simulink model "simulation"  (R2018a)
settings: Solver=VariableStepAuto  StartTime=0.0  StopTime=10.0  RelTol=1e-3
undefined symbols (not defined in the file or in its folder): booleanControl
settings Model: Creator=daniel  LastModifiedBy=daniel

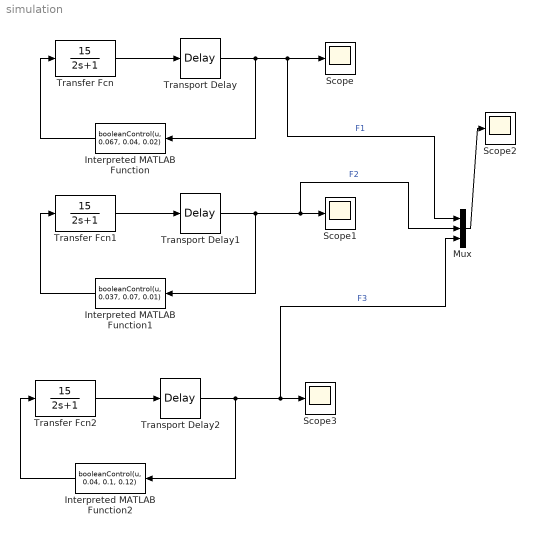
== system simulation ==
  Interpreted MATLAB Function : MATLABFcn  MATLABFcn=booleanControl(u, 0.067, 0.04, 0.02)
  Interpreted MATLAB Function1 : MATLABFcn  MATLABFcn=booleanControl(u, 0.037, 0.07, 0.01)
  Interpreted MATLAB Function2 : MATLABFcn  MATLABFcn=booleanControl(u, 0.04, 0.1, 0.12)
  Mux : Mux  Inputs=3
  Scope{,1..3} (4 alike) : Scope
  Transfer Fcn : TransferFcn  Numerator=[15]  Denominator=[2 1]
  Transfer Fcn1 : TransferFcn  Numerator=[15]  Denominator=[2 1]
  Transfer Fcn2 : TransferFcn  Numerator=[15]  Denominator=[2 1]
  Transport Delay : TransportDelay  DelayTime=0.5
  Transport Delay1 : TransportDelay  DelayTime=0.5
  Transport Delay2 : TransportDelay  DelayTime=0.5
  wires:
  Transfer Fcn/1 -> Transport Delay/1
  Transport Delay/1 -> Interpreted MATLAB Function/1, Mux/1, Scope/1  "F1"
  Interpreted MATLAB Function/1 -> Transfer Fcn/1
  Transfer Fcn1/1 -> Transport Delay1/1
  Interpreted MATLAB Function1/1 -> Transfer Fcn1/1
  Transport Delay1/1 -> Interpreted MATLAB Function1/1, Mux/2, Scope1/1  "F2"
  Mux/1 -> Scope2/1
  Transport Delay2/1 -> Interpreted MATLAB Function2/1, Mux/3, Scope3/1  "F3"
  Transfer Fcn2/1 -> Transport Delay2/1
  Interpreted MATLAB Function2/1 -> Transfer Fcn2/1
